simulink subsystem "Hauteur_Aimants_Plaque_2"  (R2021a)
settings: Solver=VariableStepAuto  StartTime=0.0  StopTime=10.0  RelTol=1e-3
settings Model: Creator=antho  LastModifiedBy=antho

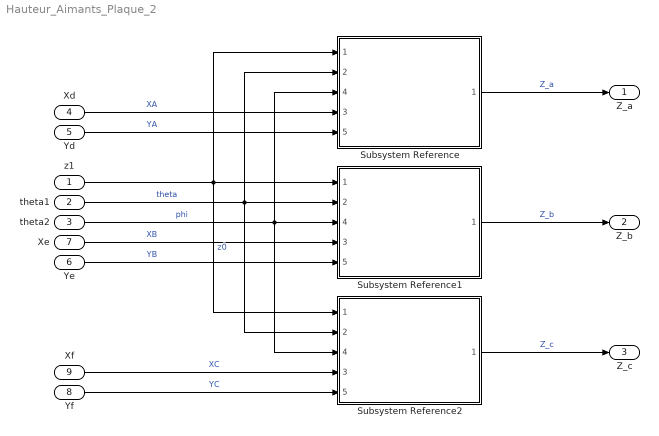
== system Hauteur_Aimants_Plaque_2 ==
  z1 : Inport
  theta1 : Inport  Port=2
  theta2 : Inport  Port=3
  Xd : Inport  Port=4
  Yd : Inport  Port=5
  Ye : Inport  Port=6
  Xe : Inport  Port=7
  Yf : Inport  Port=8
  Xf : Inport  Port=9
  Subsystem Reference : Subsystem  ReferencedSubsystem=subsys_calcul_Zk
      settings: PortSchema="{\"entries\":[{\"content\":{\"sides\":[{\"content\":{\"connectorIds\":[\"In1\",\"In2\",\"In4\",\"In3\",\"In5\"]},\"type\":\"ConnectorPlacement.EquallySpacedRectSide\",\"uuid\":\"58a7cade-cf80-43c0-946c-336fdbd8c2a7\"},{\"content\":{\"connectorIds\":[\"Out1\"],\"side\":\"RIGHT\"},\"type\":\"ConnectorPlacement.EquallySpacedRectSide\",\"uuid\":\"9a223902-f7c0-4b06-b74a-0bbf211990a4\"},{\"content\":{\"connectorIds\":[],\"side\":\"TOP\"},\"type\":\"ConnectorPlacement.EquallySpacedRectSide\",\"uuid\":\"8d5abb67-7ecf-4602-9715-44c58f718e55\"}]},\"type\":\"ConnectorPlacement.EquallySpacedConnector\",\"uuid\":\"bbfaaa32-0739-40af-9581-6fc28608cdbf\"}],\"packageUris\":[\"http://schema.mathworks.com/mf0/Connector/R2020b\"],\"version\":\"1.0\"}"
  Subsystem Reference1 : Subsystem  ReferencedSubsystem=subsys_calcul_Zk
      settings: PortSchema="{\"entries\":[{\"content\":{\"sides\":[{\"content\":{\"connectorIds\":[\"In1\",\"In2\",\"In4\",\"In3\",\"In5\"]},\"type\":\"ConnectorPlacement.EquallySpacedRectSide\",\"uuid\":\"58a7cade-cf80-43c0-946c-336fdbd8c2a7\"},{\"content\":{\"connectorIds\":[\"Out1\"],\"side\":\"RIGHT\"},\"type\":\"ConnectorPlacement.EquallySpacedRectSide\",\"uuid\":\"9a223902-f7c0-4b06-b74a-0bbf211990a4\"},{\"content\":{\"connectorIds\":[],\"side\":\"TOP\"},\"type\":\"ConnectorPlacement.EquallySpacedRectSide\",\"uuid\":\"8d5abb67-7ecf-4602-9715-44c58f718e55\"}]},\"type\":\"ConnectorPlacement.EquallySpacedConnector\",\"uuid\":\"bbfaaa32-0739-40af-9581-6fc28608cdbf\"}],\"packageUris\":[\"http://schema.mathworks.com/mf0/Connector/R2020b\"],\"version\":\"1.0\"}"
  Subsystem Reference2 : Subsystem  ReferencedSubsystem=subsys_calcul_Zk
      settings: PortSchema="{\"entries\":[{\"content\":{\"sides\":[{\"content\":{\"connectorIds\":[\"In1\",\"In2\",\"In4\",\"In3\",\"In5\"]},\"type\":\"ConnectorPlacement.EquallySpacedRectSide\",\"uuid\":\"58a7cade-cf80-43c0-946c-336fdbd8c2a7\"},{\"content\":{\"connectorIds\":[\"Out1\"],\"side\":\"RIGHT\"},\"type\":\"ConnectorPlacement.EquallySpacedRectSide\",\"uuid\":\"9a223902-f7c0-4b06-b74a-0bbf211990a4\"},{\"content\":{\"connectorIds\":[],\"side\":\"TOP\"},\"type\":\"ConnectorPlacement.EquallySpacedRectSide\",\"uuid\":\"8d5abb67-7ecf-4602-9715-44c58f718e55\"}]},\"type\":\"ConnectorPlacement.EquallySpacedConnector\",\"uuid\":\"bbfaaa32-0739-40af-9581-6fc28608cdbf\"}],\"packageUris\":[\"http://schema.mathworks.com/mf0/Connector/R2020b\"],\"version\":\"1.0\"}"
  Z_a : Outport
  Z_b : Outport  Port=2
  Z_c : Outport  Port=3
  wires:
  Subsystem Reference2/1 -> Z_c/1  "Z_c"
  Subsystem Reference/1 -> Z_a/1  "Z_a"
  Subsystem Reference1/1 -> Z_b/1  "Z_b"
  z1/1 -> Subsystem Reference1/1, Subsystem Reference/1, Subsystem Reference2/1  "z0"
  theta2/1 -> Subsystem Reference2/4, Subsystem Reference1/4, Subsystem Reference/4  "phi"
  theta1/1 -> Subsystem Reference1/2, Subsystem Reference/2, Subsystem Reference2/2  "theta"
  Yd/1 -> Subsystem Reference/5  "YA"
  Xd/1 -> Subsystem Reference/3  "XA"
  Xe/1 -> Subsystem Reference1/3  "XB"
  Ye/1 -> Subsystem Reference1/5  "YB"
  Xf/1 -> Subsystem Reference2/3  "XC"
  Yf/1 -> Subsystem Reference2/5  "YC"
